simulink model "simulate_inv_dyn_2dofplanar"  (Simulink 8.5)
settings: Solver=ode3  StartTime=0.0  StopTime=10  FixedStep=0.01  MaxStep=0.001  MinStep=0.0005  RelTol=1e-3
undefined symbols (not defined in the file or in its folder): call_inverse_dynamics
settings Model: Creator=arturo  LastModifiedBy=arturogilaparicio
settings DebuggingCC: SolverPrmCheckMsg=warning  FcnCallInpInsideContextMsg=UseLocalSettings

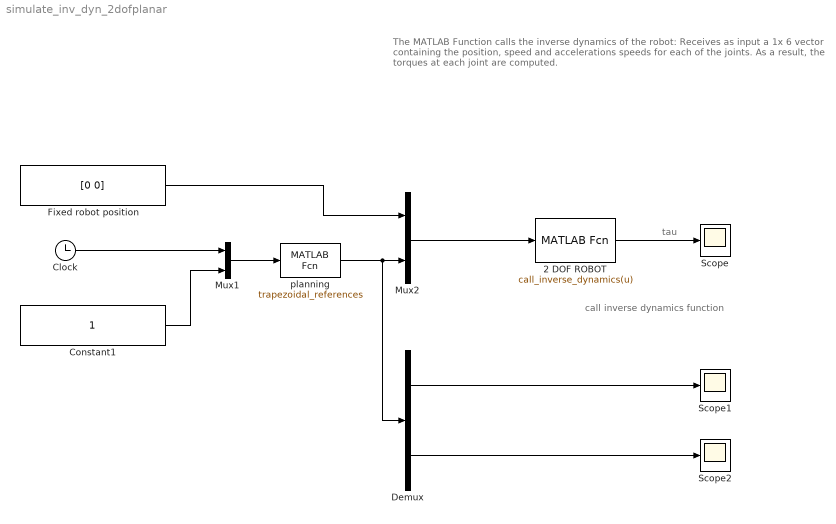
== system simulate_inv_dyn_2dofplanar ==
  note: tau
  note: The MATLAB Function calls the inverse dynamics of the robot:
      | Receives as input a 1x 6 vector containing the
      | position, speed and accelerations
      | speeds for each of the joints. As a result, the torques at each joint are computed.
  note: call inverse dynamics
      |  function
  2 DOF ROBOT : MATLABFcn  MATLABFcn=call_inverse_dynamics(u)  OutputDimensions=2
  Clock : Clock
  Constant1 : Constant
  Demux : Demux  Outputs=2
  Fixed robot position : Constant  Value=[0 0]
  Mux1 : Mux  Inputs=2
  Mux2 : Mux  Inputs=2
  Scope : Scope
      settings: YMin=-500  YMax=200
  Scope1 : Scope
      settings: YMin=1.65806  YMax=1.8326
  Scope2 : Scope
      settings: YMin=-500  YMax=200  SaveName=ScopeData2
  planning : MATLABFcn  MATLABFcn=trapezoidal_references  OutputDimensions=4
  wires:
  Mux2/1 -> 2 DOF ROBOT/1
  2 DOF ROBOT/1 -> Scope/1
  Fixed robot position/1 -> Mux2/1
  Mux1/1 -> planning/1
  Clock/1 -> Mux1/1
  Constant1/1 -> Mux1/2
  planning/1 -> Demux/1, Mux2/2
  Demux/1 -> Scope1/1
  Demux/2 -> Scope2/1
